simulink model "iir_original"  (R2024b)
settings: Solver=FixedStepDiscrete  StartTime=0.0  StopTime=10.0  FixedStep=Ts  RelTol=1e-3
PreLoadFcn:
  | if ~exist('b','var'), iir_setup; end
values from neighbouring files (symbols this model uses):
  Ts = 1/Fs    (= 2.08333333333e-05)    [iir_setup.m]
undefined symbols (not defined in the file or in its folder): a, b
settings Model: Creator=samue  LastModifiedBy=samue
settings DataIOCC: SaveTime=off
settings DebuggingCC: ParameterPrecisionLossMsg=none

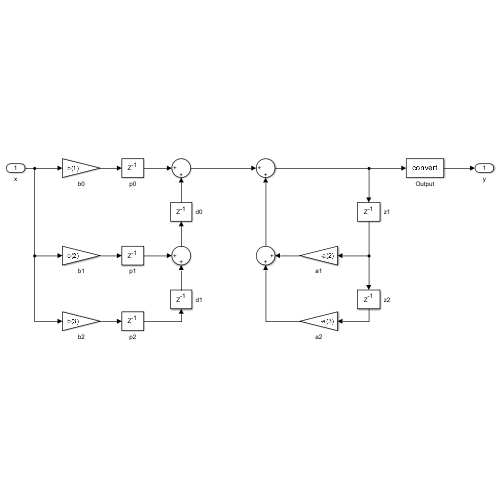
[thumbnail: Simulink's stored preview of the top-level diagram]
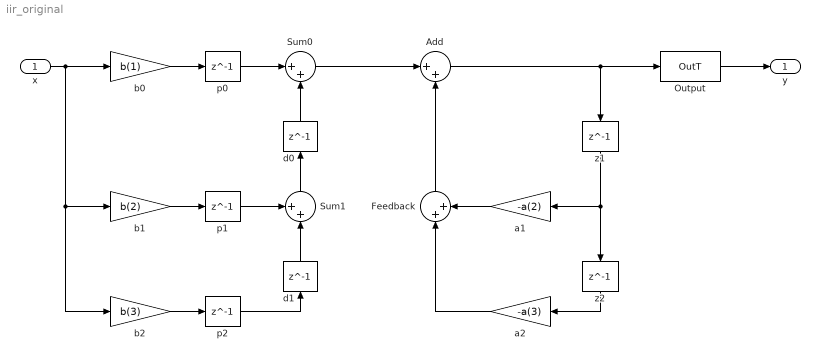
== system iir_original ==
  x : Inport  OutDataTypeStr=InT  SampleTime=Ts
  Add : Sum  Inputs=|++  OutDataTypeStr=SigT
  Feedback : Sum  Inputs=|++  OutDataTypeStr=SigT
  Output : DataTypeConversion  OutDataTypeStr=OutT  RndMeth=Floor
  Sum0 : Sum  Inputs=|++  OutDataTypeStr=SigT
  Sum1 : Sum  Inputs=++|  OutDataTypeStr=SigT
  a1 : Gain  Gain=-a(2)  ParamDataTypeStr=fixdt(1,CoeffWL)  OutDataTypeStr=SigT
  a2 : Gain  Gain=-a(3)  ParamDataTypeStr=fixdt(1,CoeffWL)  OutDataTypeStr=SigT
  b0 : Gain  Gain=b(1)  ParamDataTypeStr=fixdt(1,CoeffWL)  OutDataTypeStr=SigT
  b1 : Gain  Gain=b(2)  ParamDataTypeStr=fixdt(1,CoeffWL)  OutDataTypeStr=SigT
  b2 : Gain  Gain=b(3)  ParamDataTypeStr=fixdt(1,CoeffWL)  OutDataTypeStr=SigT
  d0 : Delay  DelayLength=1
  d1 : Delay  DelayLength=1
  p0 : Delay  DelayLength=1
  p1 : Delay  DelayLength=1
  p2 : Delay  DelayLength=1
  z1 : Delay  DelayLength=1
  z2 : Delay  DelayLength=1
  y : Outport
  wires:
  x/1 -> b1/1, b2/1, b0/1
  b0/1 -> p0/1
  b1/1 -> p1/1
  b2/1 -> p2/1
  p0/1 -> Sum0/1
  d0/1 -> Sum0/2
  p1/1 -> Sum1/1
  d1/1 -> Sum1/2
  Sum1/1 -> d0/1
  p2/1 -> d1/1
  Sum0/1 -> Add/1
  Add/1 -> Output/1, z1/1
  Output/1 -> y/1
  z1/1 -> z2/1, a1/1
  z2/1 -> a2/1
  a1/1 -> Feedback/2
  a2/1 -> Feedback/1
  Feedback/1 -> Add/2
